simulink model "dvoupatrak_15lan"  (R2019b)
settings: Solver=VariableStepAuto  StartTime=0.0  StopTime=sim_time  RelTol=1e-3  AbsTol=1e-3
InitFcn:
  | parameters_dvoupatrak;
values from neighbouring files (symbols this model uses):
  b_d = b_diameter * ones(6,1)    [parameters_dvoupatrak.m]
  b_l = b_length * ones(6,1)    [parameters_dvoupatrak.m]
  b_rho = b_density * ones(6,1)    [parameters_dvoupatrak.m]
  bp = bpi * ones(15,1)    [parameters_dvoupatrak.m]
  bs = c_specific_damping * ones(15,1)    [parameters_dvoupatrak.m]
  kp = kpi * ones(15,1)    [parameters_dvoupatrak.m]
  ks = c_specific_stiffness * ones(15,1)    [parameters_dvoupatrak.m]
  l0_init = cable_length(node_coords, incidence_table(7:end,:))    [parameters_dvoupatrak.m]
  N = node_coords    [parameters_dvoupatrak.m]
  prestress_cab = 0.95    [simulate.m]
  r_mid = 0.15    [parameters_dvoupatrak.m]
  settling_time = 0.5    [simulate.m]
  sim_time = 5    [simulate.m]
  v1 = sqrt(b_length^2 - (xB-xA)^2 - (yB-yA)^2)    [parameters_dvoupatrak.m]
  v2 = sqrt(b_length^2 - (xC-xB)^2 - (yC-yB)^2)    [parameters_dvoupatrak.m]
undefined symbols (not defined in the file or in its folder): X, Y, Z
libraries: nesl_utility x88, sm_lib x70, cstblocks x15, simulink x8
(part 3 of 4)

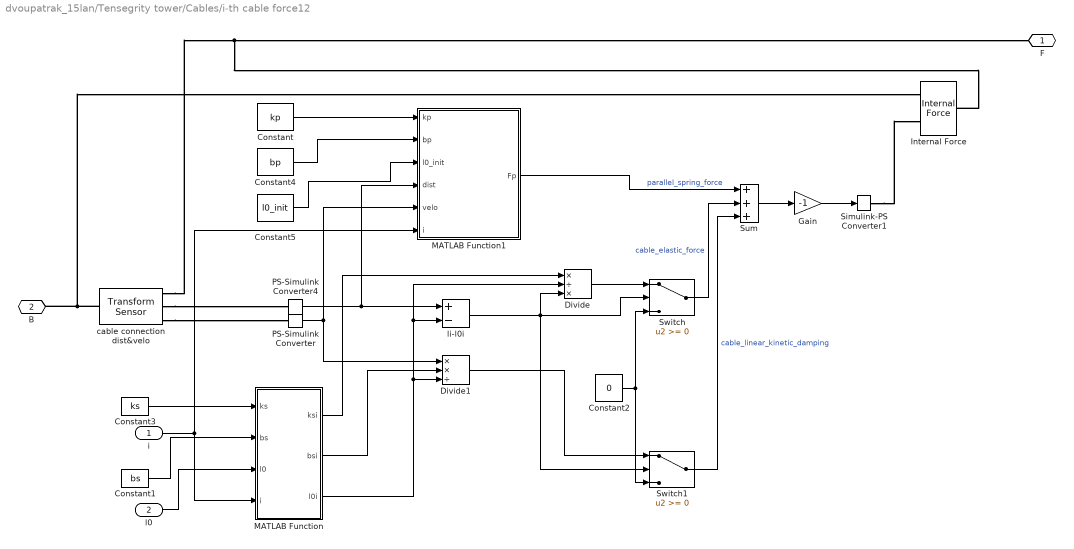
== system dvoupatrak_15lan/Tensegrity tower/Cables/i-th cable force12 ==
  i : Inport
  l0 : Inport  Port=2
  Constant : Constant  Value=kp
  Constant1 : Constant  Value=bs
  Constant2 : Constant  Value=0
  Constant3 : Constant  Value=ks
  Constant4 : Constant  Value=bp
  Constant5 : Constant  Value=l0_init
  Divide : Product  Inputs=*/*
  Divide1 : Product  Inputs=**/
  Gain : Gain  Gain=-1
  Internal Force : sm_lib/Forces and Torques/Internal Force
      settings: SourceProductBaseCode=MS
  MATLAB Function : MATLAB Function  TreatAsAtomicUnit=on
  MATLAB Function1 : MATLAB Function  TreatAsAtomicUnit=on
  PS-Simulink Converter : nesl_utility/PS-Simulink Converter  PhysicalDomain=network_engine_domain  SubClassName=ps_output  LeftPortType=input  RightPortType=output  PseudoPeriodic=off  Frequencies=[]  Unit=inherit  AffineConversion=off
  PS-Simulink Converter4 : nesl_utility/PS-Simulink Converter  PhysicalDomain=network_engine_domain  SubClassName=ps_output  LeftPortType=input  RightPortType=output  PseudoPeriodic=off  Frequencies=[]  Unit=inherit  AffineConversion=off
  Simulink-PS Converter1 : nesl_utility/Simulink-PS Converter  PhysicalDomain=network_engine_domain  SubClassName=ps_input  LeftPortType=input  RightPortType=output  PseudoPeriodic=off  Frequencies=[]  NoiseDistribution=none  NoiseParameters=[]  Unit=1  AffineConversion=off  FilteringAndDerivatives=provide  SimscapeFilterOrder=1  InputFilterTimeConstant=0.001  UdotUserProvided=0
  Sum : Sum  Inputs=+++
  Switch : Switch
  Switch1 : Switch
  cable connection dist&velo : sm_lib/Frames and Transforms/Transform Sensor  MeasurementFrame=World  SenseAngle=off  SenseAxis=off  SenseAngle1=off  SenseAngle2=off  SenseAngle3=off  SenseQ=off  SenseR=off  SenseOmegaX=off  SenseOmegaY=off  SenseOmegaZ=off  SenseOmega1=off  SenseOmega2=off  SenseOmega3=off  SenseQDot=off  SenseRDot=off  SenseAlphaX=off  SenseAlphaY=off  SenseAlphaZ=off  SenseAlpha1=off  SenseAlpha2=off  SenseAlpha3=off  SenseQDDot=off  SenseRDDot=off  SenseX=off  SenseY=off  SenseZ=off  SenseRad=off  SenseAzim=off  SenseDist=on  SenseInc=off  SenseXDot=off  SenseYDot=off  SenseZDot=off  SenseRadDot=off  SenseAzimDot=off  SenseDistDot=on  SenseIncDot=off  SenseXDDot=off  SenseYDDot=off  SenseZDDot=off  SenseRadDDot=off  SenseAzimDDot=off  SenseDistDDot=off  SenseIncDDot=off
  li-l0i : Sum  Inputs=+-
  F : PMIOPort  Side=Right
  B : PMIOPort  Port=2  Side=Left
  wires:
  Constant1/1 -> MATLAB Function/2(bs)
  Switch1/1 -> Sum/3  "cable_linear_kinetic_damping"
  Divide/1 -> Switch/1
  Switch/1 -> Sum/2  "cable_elastic_force"
  MATLAB Function/2(bsi) -> Divide1/2
  Constant3/1 -> MATLAB Function/1(ks)
  Divide1/1 -> Switch1/1
  MATLAB Function/1(ksi) -> Divide/1
  Constant/1 -> MATLAB Function1/1(kp)
  Constant4/1 -> MATLAB Function1/2(bp)
  Constant5/1 -> MATLAB Function1/3(l0_init)
  MATLAB Function1/1(Fp) -> Sum/1  "parallel_spring_force"
  Sum/1 -> Gain/1
  Gain/1 -> Simulink-PS Converter1/1
  li-l0i/1 -> Switch/2, Divide/3, Switch1/2
  l0/1 -> MATLAB Function/3(l0)
  Constant2/1 -> Switch1/3, Switch/3
  MATLAB Function/3(l0i) -> Divide1/3, Divide/2, li-l0i/2
  PS-Simulink Converter4/1 -> li-l0i/1, MATLAB Function1/4(dist)
  PS-Simulink Converter/1 -> Divide1/1, MATLAB Function1/5(velo)
  i/1 -> MATLAB Function/4(i), MATLAB Function1/6(i)
  connections:
  cable connection dist&velo/RConn3 -- PS-Simulink Converter/LConn1
  cable connection dist&velo/RConn1 -- Internal Force/RConn1 -- F/RConn1
  cable connection dist&velo/RConn2 -- PS-Simulink Converter4/LConn1
  Simulink-PS Converter1/RConn1 -- Internal Force/LConn2
  cable connection dist&velo/LConn1 -- B/RConn1 -- Internal Force/LConn1

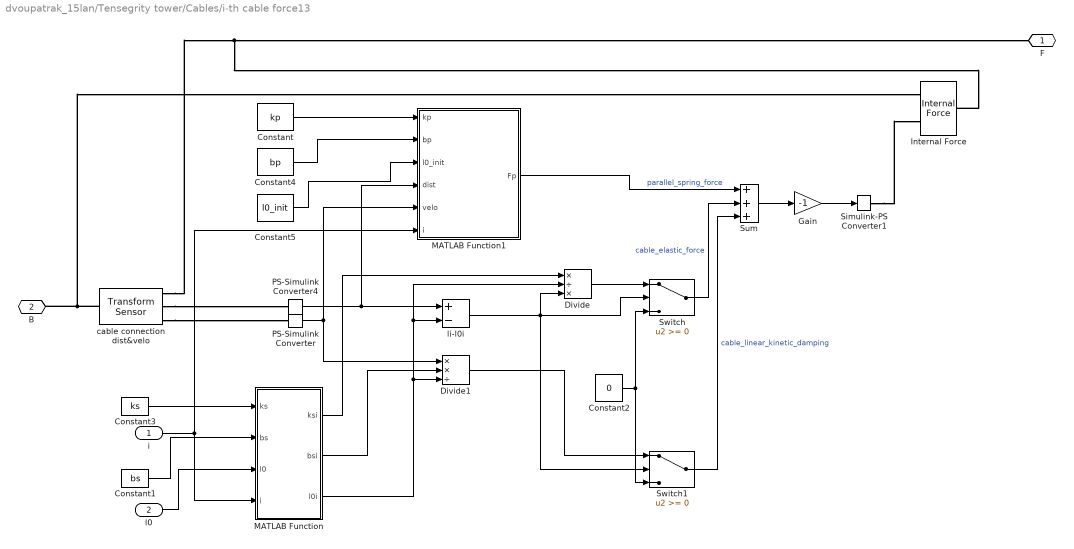
== system dvoupatrak_15lan/Tensegrity tower/Cables/i-th cable force13 ==
  i : Inport
  l0 : Inport  Port=2
  Constant : Constant  Value=kp
  Constant1 : Constant  Value=bs
  Constant2 : Constant  Value=0
  Constant3 : Constant  Value=ks
  Constant4 : Constant  Value=bp
  Constant5 : Constant  Value=l0_init
  Divide : Product  Inputs=*/*
  Divide1 : Product  Inputs=**/
  Gain : Gain  Gain=-1
  Internal Force : sm_lib/Forces and Torques/Internal Force
      settings: SourceProductBaseCode=MS
  MATLAB Function : MATLAB Function  TreatAsAtomicUnit=on
  MATLAB Function1 : MATLAB Function  TreatAsAtomicUnit=on
  PS-Simulink Converter : nesl_utility/PS-Simulink Converter  PhysicalDomain=network_engine_domain  SubClassName=ps_output  LeftPortType=input  RightPortType=output  PseudoPeriodic=off  Frequencies=[]  Unit=inherit  AffineConversion=off
  PS-Simulink Converter4 : nesl_utility/PS-Simulink Converter  PhysicalDomain=network_engine_domain  SubClassName=ps_output  LeftPortType=input  RightPortType=output  PseudoPeriodic=off  Frequencies=[]  Unit=inherit  AffineConversion=off
  Simulink-PS Converter1 : nesl_utility/Simulink-PS Converter  PhysicalDomain=network_engine_domain  SubClassName=ps_input  LeftPortType=input  RightPortType=output  PseudoPeriodic=off  Frequencies=[]  NoiseDistribution=none  NoiseParameters=[]  Unit=1  AffineConversion=off  FilteringAndDerivatives=provide  SimscapeFilterOrder=1  InputFilterTimeConstant=0.001  UdotUserProvided=0
  Sum : Sum  Inputs=+++
  Switch : Switch
  Switch1 : Switch
  cable connection dist&velo : sm_lib/Frames and Transforms/Transform Sensor  MeasurementFrame=World  SenseAngle=off  SenseAxis=off  SenseAngle1=off  SenseAngle2=off  SenseAngle3=off  SenseQ=off  SenseR=off  SenseOmegaX=off  SenseOmegaY=off  SenseOmegaZ=off  SenseOmega1=off  SenseOmega2=off  SenseOmega3=off  SenseQDot=off  SenseRDot=off  SenseAlphaX=off  SenseAlphaY=off  SenseAlphaZ=off  SenseAlpha1=off  SenseAlpha2=off  SenseAlpha3=off  SenseQDDot=off  SenseRDDot=off  SenseX=off  SenseY=off  SenseZ=off  SenseRad=off  SenseAzim=off  SenseDist=on  SenseInc=off  SenseXDot=off  SenseYDot=off  SenseZDot=off  SenseRadDot=off  SenseAzimDot=off  SenseDistDot=on  SenseIncDot=off  SenseXDDot=off  SenseYDDot=off  SenseZDDot=off  SenseRadDDot=off  SenseAzimDDot=off  SenseDistDDot=off  SenseIncDDot=off
  li-l0i : Sum  Inputs=+-
  F : PMIOPort  Side=Right
  B : PMIOPort  Port=2  Side=Left
  wires:
  Constant1/1 -> MATLAB Function/2(bs)
  Switch1/1 -> Sum/3  "cable_linear_kinetic_damping"
  Divide/1 -> Switch/1
  Switch/1 -> Sum/2  "cable_elastic_force"
  MATLAB Function/2(bsi) -> Divide1/2
  Constant3/1 -> MATLAB Function/1(ks)
  Divide1/1 -> Switch1/1
  MATLAB Function/1(ksi) -> Divide/1
  Constant/1 -> MATLAB Function1/1(kp)
  Constant4/1 -> MATLAB Function1/2(bp)
  Constant5/1 -> MATLAB Function1/3(l0_init)
  MATLAB Function1/1(Fp) -> Sum/1  "parallel_spring_force"
  Sum/1 -> Gain/1
  Gain/1 -> Simulink-PS Converter1/1
  li-l0i/1 -> Switch/2, Divide/3, Switch1/2
  l0/1 -> MATLAB Function/3(l0)
  Constant2/1 -> Switch1/3, Switch/3
  MATLAB Function/3(l0i) -> Divide1/3, Divide/2, li-l0i/2
  PS-Simulink Converter4/1 -> li-l0i/1, MATLAB Function1/4(dist)
  PS-Simulink Converter/1 -> Divide1/1, MATLAB Function1/5(velo)
  i/1 -> MATLAB Function/4(i), MATLAB Function1/6(i)
  connections:
  cable connection dist&velo/RConn3 -- PS-Simulink Converter/LConn1
  cable connection dist&velo/RConn1 -- Internal Force/RConn1 -- F/RConn1
  cable connection dist&velo/RConn2 -- PS-Simulink Converter4/LConn1
  Simulink-PS Converter1/RConn1 -- Internal Force/LConn2
  cable connection dist&velo/LConn1 -- B/RConn1 -- Internal Force/LConn1

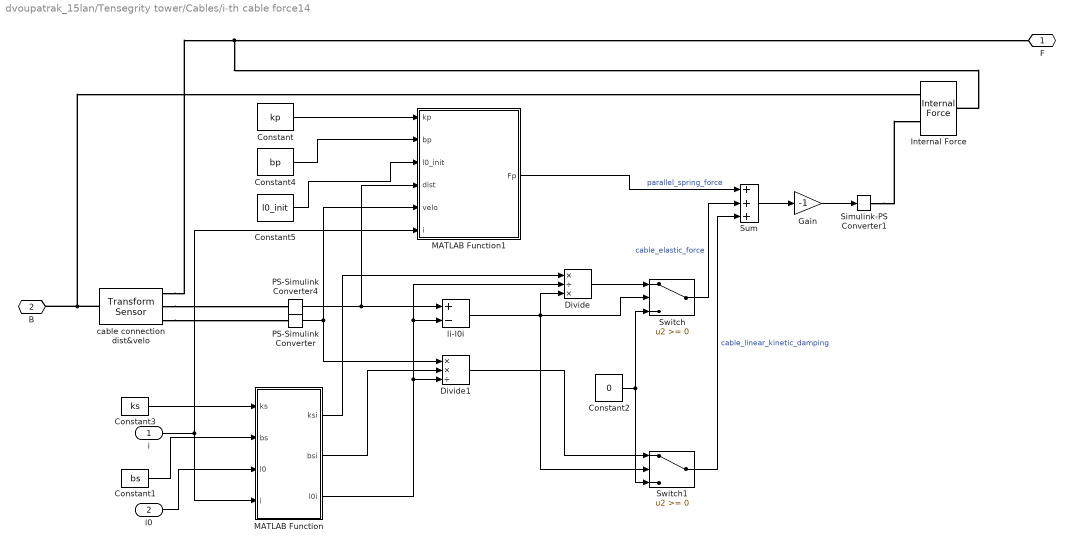
== system dvoupatrak_15lan/Tensegrity tower/Cables/i-th cable force14 ==
  i : Inport
  l0 : Inport  Port=2
  Constant : Constant  Value=kp
  Constant1 : Constant  Value=bs
  Constant2 : Constant  Value=0
  Constant3 : Constant  Value=ks
  Constant4 : Constant  Value=bp
  Constant5 : Constant  Value=l0_init
  Divide : Product  Inputs=*/*
  Divide1 : Product  Inputs=**/
  Gain : Gain  Gain=-1
  Internal Force : sm_lib/Forces and Torques/Internal Force
      settings: SourceProductBaseCode=MS
  MATLAB Function : MATLAB Function  TreatAsAtomicUnit=on
  MATLAB Function1 : MATLAB Function  TreatAsAtomicUnit=on
  PS-Simulink Converter : nesl_utility/PS-Simulink Converter  PhysicalDomain=network_engine_domain  SubClassName=ps_output  LeftPortType=input  RightPortType=output  PseudoPeriodic=off  Frequencies=[]  Unit=inherit  AffineConversion=off
  PS-Simulink Converter4 : nesl_utility/PS-Simulink Converter  PhysicalDomain=network_engine_domain  SubClassName=ps_output  LeftPortType=input  RightPortType=output  PseudoPeriodic=off  Frequencies=[]  Unit=inherit  AffineConversion=off
  Simulink-PS Converter1 : nesl_utility/Simulink-PS Converter  PhysicalDomain=network_engine_domain  SubClassName=ps_input  LeftPortType=input  RightPortType=output  PseudoPeriodic=off  Frequencies=[]  NoiseDistribution=none  NoiseParameters=[]  Unit=1  AffineConversion=off  FilteringAndDerivatives=provide  SimscapeFilterOrder=1  InputFilterTimeConstant=0.001  UdotUserProvided=0
  Sum : Sum  Inputs=+++
  Switch : Switch
  Switch1 : Switch
  cable connection dist&velo : sm_lib/Frames and Transforms/Transform Sensor  MeasurementFrame=World  SenseAngle=off  SenseAxis=off  SenseAngle1=off  SenseAngle2=off  SenseAngle3=off  SenseQ=off  SenseR=off  SenseOmegaX=off  SenseOmegaY=off  SenseOmegaZ=off  SenseOmega1=off  SenseOmega2=off  SenseOmega3=off  SenseQDot=off  SenseRDot=off  SenseAlphaX=off  SenseAlphaY=off  SenseAlphaZ=off  SenseAlpha1=off  SenseAlpha2=off  SenseAlpha3=off  SenseQDDot=off  SenseRDDot=off  SenseX=off  SenseY=off  SenseZ=off  SenseRad=off  SenseAzim=off  SenseDist=on  SenseInc=off  SenseXDot=off  SenseYDot=off  SenseZDot=off  SenseRadDot=off  SenseAzimDot=off  SenseDistDot=on  SenseIncDot=off  SenseXDDot=off  SenseYDDot=off  SenseZDDot=off  SenseRadDDot=off  SenseAzimDDot=off  SenseDistDDot=off  SenseIncDDot=off
  li-l0i : Sum  Inputs=+-
  F : PMIOPort  Side=Right
  B : PMIOPort  Port=2  Side=Left
  wires:
  Constant1/1 -> MATLAB Function/2(bs)
  Switch1/1 -> Sum/3  "cable_linear_kinetic_damping"
  Divide/1 -> Switch/1
  Switch/1 -> Sum/2  "cable_elastic_force"
  MATLAB Function/2(bsi) -> Divide1/2
  Constant3/1 -> MATLAB Function/1(ks)
  Divide1/1 -> Switch1/1
  MATLAB Function/1(ksi) -> Divide/1
  Constant/1 -> MATLAB Function1/1(kp)
  Constant4/1 -> MATLAB Function1/2(bp)
  Constant5/1 -> MATLAB Function1/3(l0_init)
  MATLAB Function1/1(Fp) -> Sum/1  "parallel_spring_force"
  Sum/1 -> Gain/1
  Gain/1 -> Simulink-PS Converter1/1
  li-l0i/1 -> Switch/2, Divide/3, Switch1/2
  l0/1 -> MATLAB Function/3(l0)
  Constant2/1 -> Switch1/3, Switch/3
  MATLAB Function/3(l0i) -> Divide1/3, Divide/2, li-l0i/2
  PS-Simulink Converter4/1 -> li-l0i/1, MATLAB Function1/4(dist)
  PS-Simulink Converter/1 -> Divide1/1, MATLAB Function1/5(velo)
  i/1 -> MATLAB Function/4(i), MATLAB Function1/6(i)
  connections:
  cable connection dist&velo/RConn3 -- PS-Simulink Converter/LConn1
  cable connection dist&velo/RConn1 -- Internal Force/RConn1 -- F/RConn1
  cable connection dist&velo/RConn2 -- PS-Simulink Converter4/LConn1
  Simulink-PS Converter1/RConn1 -- Internal Force/LConn2
  cable connection dist&velo/LConn1 -- B/RConn1 -- Internal Force/LConn1

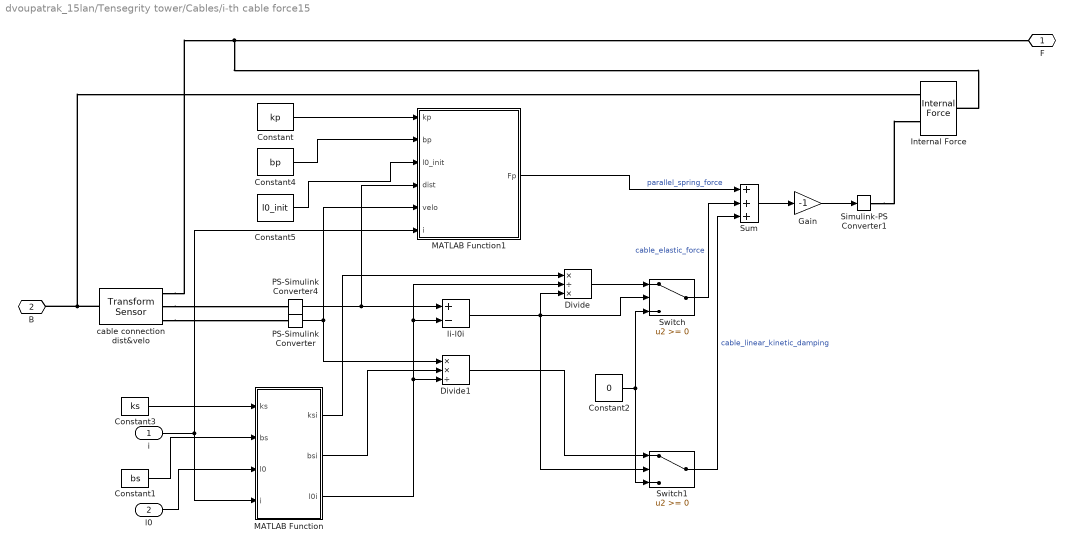
== system dvoupatrak_15lan/Tensegrity tower/Cables/i-th cable force15 ==
  i : Inport
  l0 : Inport  Port=2
  Constant : Constant  Value=kp
  Constant1 : Constant  Value=bs
  Constant2 : Constant  Value=0
  Constant3 : Constant  Value=ks
  Constant4 : Constant  Value=bp
  Constant5 : Constant  Value=l0_init
  Divide : Product  Inputs=*/*
  Divide1 : Product  Inputs=**/
  Gain : Gain  Gain=-1
  Internal Force : sm_lib/Forces and Torques/Internal Force
      settings: SourceProductBaseCode=MS
  MATLAB Function : MATLAB Function  TreatAsAtomicUnit=on
  MATLAB Function1 : MATLAB Function  TreatAsAtomicUnit=on
  PS-Simulink Converter : nesl_utility/PS-Simulink Converter  PhysicalDomain=network_engine_domain  SubClassName=ps_output  LeftPortType=input  RightPortType=output  PseudoPeriodic=off  Frequencies=[]  Unit=inherit  AffineConversion=off
  PS-Simulink Converter4 : nesl_utility/PS-Simulink Converter  PhysicalDomain=network_engine_domain  SubClassName=ps_output  LeftPortType=input  RightPortType=output  PseudoPeriodic=off  Frequencies=[]  Unit=inherit  AffineConversion=off
  Simulink-PS Converter1 : nesl_utility/Simulink-PS Converter  PhysicalDomain=network_engine_domain  SubClassName=ps_input  LeftPortType=input  RightPortType=output  PseudoPeriodic=off  Frequencies=[]  NoiseDistribution=none  NoiseParameters=[]  Unit=1  AffineConversion=off  FilteringAndDerivatives=provide  SimscapeFilterOrder=1  InputFilterTimeConstant=0.001  UdotUserProvided=0
  Sum : Sum  Inputs=+++
  Switch : Switch
  Switch1 : Switch
  cable connection dist&velo : sm_lib/Frames and Transforms/Transform Sensor  MeasurementFrame=World  SenseAngle=off  SenseAxis=off  SenseAngle1=off  SenseAngle2=off  SenseAngle3=off  SenseQ=off  SenseR=off  SenseOmegaX=off  SenseOmegaY=off  SenseOmegaZ=off  SenseOmega1=off  SenseOmega2=off  SenseOmega3=off  SenseQDot=off  SenseRDot=off  SenseAlphaX=off  SenseAlphaY=off  SenseAlphaZ=off  SenseAlpha1=off  SenseAlpha2=off  SenseAlpha3=off  SenseQDDot=off  SenseRDDot=off  SenseX=off  SenseY=off  SenseZ=off  SenseRad=off  SenseAzim=off  SenseDist=on  SenseInc=off  SenseXDot=off  SenseYDot=off  SenseZDot=off  SenseRadDot=off  SenseAzimDot=off  SenseDistDot=on  SenseIncDot=off  SenseXDDot=off  SenseYDDot=off  SenseZDDot=off  SenseRadDDot=off  SenseAzimDDot=off  SenseDistDDot=off  SenseIncDDot=off
  li-l0i : Sum  Inputs=+-
  F : PMIOPort  Side=Right
  B : PMIOPort  Port=2  Side=Left
  wires:
  Constant1/1 -> MATLAB Function/2(bs)
  Switch1/1 -> Sum/3  "cable_linear_kinetic_damping"
  Divide/1 -> Switch/1
  Switch/1 -> Sum/2  "cable_elastic_force"
  MATLAB Function/2(bsi) -> Divide1/2
  Constant3/1 -> MATLAB Function/1(ks)
  Divide1/1 -> Switch1/1
  MATLAB Function/1(ksi) -> Divide/1
  Constant/1 -> MATLAB Function1/1(kp)
  Constant4/1 -> MATLAB Function1/2(bp)
  Constant5/1 -> MATLAB Function1/3(l0_init)
  MATLAB Function1/1(Fp) -> Sum/1  "parallel_spring_force"
  Sum/1 -> Gain/1
  Gain/1 -> Simulink-PS Converter1/1
  li-l0i/1 -> Switch/2, Divide/3, Switch1/2
  l0/1 -> MATLAB Function/3(l0)
  Constant2/1 -> Switch1/3, Switch/3
  MATLAB Function/3(l0i) -> Divide1/3, Divide/2, li-l0i/2
  PS-Simulink Converter4/1 -> li-l0i/1, MATLAB Function1/4(dist)
  PS-Simulink Converter/1 -> Divide1/1, MATLAB Function1/5(velo)
  i/1 -> MATLAB Function/4(i), MATLAB Function1/6(i)
  connections:
  cable connection dist&velo/RConn3 -- PS-Simulink Converter/LConn1
  cable connection dist&velo/RConn1 -- Internal Force/RConn1 -- F/RConn1
  cable connection dist&velo/RConn2 -- PS-Simulink Converter4/LConn1
  Simulink-PS Converter1/RConn1 -- Internal Force/LConn2
  cable connection dist&velo/LConn1 -- B/RConn1 -- Internal Force/LConn1

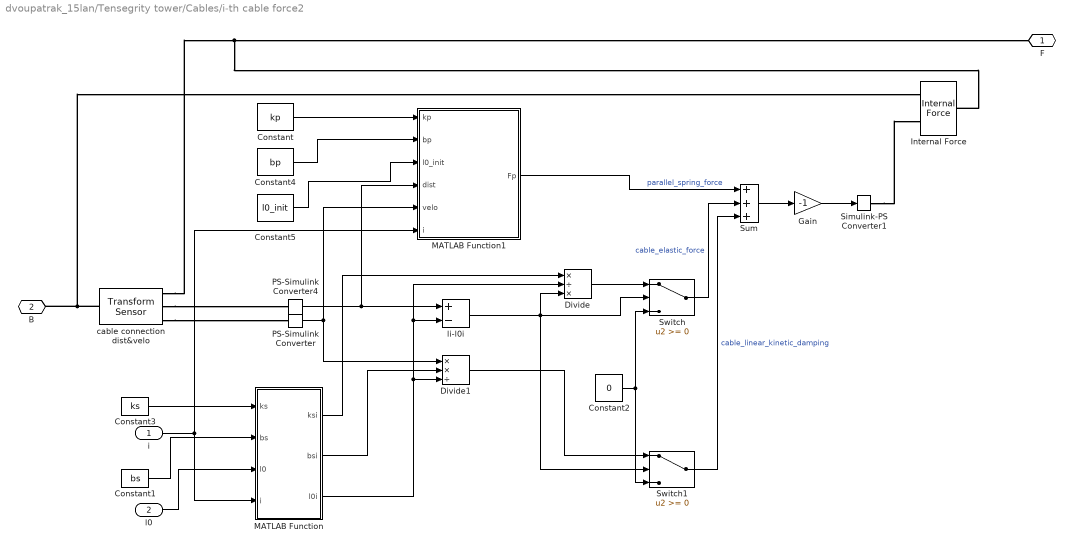
== system dvoupatrak_15lan/Tensegrity tower/Cables/i-th cable force2 ==
  i : Inport
  l0 : Inport  Port=2
  Constant : Constant  Value=kp
  Constant1 : Constant  Value=bs
  Constant2 : Constant  Value=0
  Constant3 : Constant  Value=ks
  Constant4 : Constant  Value=bp
  Constant5 : Constant  Value=l0_init
  Divide : Product  Inputs=*/*
  Divide1 : Product  Inputs=**/
  Gain : Gain  Gain=-1
  Internal Force : sm_lib/Forces and Torques/Internal Force
      settings: SourceProductBaseCode=MS
  MATLAB Function : MATLAB Function  TreatAsAtomicUnit=on
  MATLAB Function1 : MATLAB Function  TreatAsAtomicUnit=on
  PS-Simulink Converter : nesl_utility/PS-Simulink Converter  PhysicalDomain=network_engine_domain  SubClassName=ps_output  LeftPortType=input  RightPortType=output  PseudoPeriodic=off  Frequencies=[]  Unit=inherit  AffineConversion=off
  PS-Simulink Converter4 : nesl_utility/PS-Simulink Converter  PhysicalDomain=network_engine_domain  SubClassName=ps_output  LeftPortType=input  RightPortType=output  PseudoPeriodic=off  Frequencies=[]  Unit=inherit  AffineConversion=off
  Simulink-PS Converter1 : nesl_utility/Simulink-PS Converter  PhysicalDomain=network_engine_domain  SubClassName=ps_input  LeftPortType=input  RightPortType=output  PseudoPeriodic=off  Frequencies=[]  NoiseDistribution=none  NoiseParameters=[]  Unit=1  AffineConversion=off  FilteringAndDerivatives=provide  SimscapeFilterOrder=1  InputFilterTimeConstant=0.001  UdotUserProvided=0
  Sum : Sum  Inputs=+++
  Switch : Switch
  Switch1 : Switch
  cable connection dist&velo : sm_lib/Frames and Transforms/Transform Sensor  MeasurementFrame=World  SenseAngle=off  SenseAxis=off  SenseAngle1=off  SenseAngle2=off  SenseAngle3=off  SenseQ=off  SenseR=off  SenseOmegaX=off  SenseOmegaY=off  SenseOmegaZ=off  SenseOmega1=off  SenseOmega2=off  SenseOmega3=off  SenseQDot=off  SenseRDot=off  SenseAlphaX=off  SenseAlphaY=off  SenseAlphaZ=off  SenseAlpha1=off  SenseAlpha2=off  SenseAlpha3=off  SenseQDDot=off  SenseRDDot=off  SenseX=off  SenseY=off  SenseZ=off  SenseRad=off  SenseAzim=off  SenseDist=on  SenseInc=off  SenseXDot=off  SenseYDot=off  SenseZDot=off  SenseRadDot=off  SenseAzimDot=off  SenseDistDot=on  SenseIncDot=off  SenseXDDot=off  SenseYDDot=off  SenseZDDot=off  SenseRadDDot=off  SenseAzimDDot=off  SenseDistDDot=off  SenseIncDDot=off
  li-l0i : Sum  Inputs=+-
  F : PMIOPort  Side=Right
  B : PMIOPort  Port=2  Side=Left
  wires:
  Constant1/1 -> MATLAB Function/2(bs)
  Switch1/1 -> Sum/3  "cable_linear_kinetic_damping"
  Divide/1 -> Switch/1
  Switch/1 -> Sum/2  "cable_elastic_force"
  MATLAB Function/2(bsi) -> Divide1/2
  Constant3/1 -> MATLAB Function/1(ks)
  Divide1/1 -> Switch1/1
  MATLAB Function/1(ksi) -> Divide/1
  Constant/1 -> MATLAB Function1/1(kp)
  Constant4/1 -> MATLAB Function1/2(bp)
  Constant5/1 -> MATLAB Function1/3(l0_init)
  MATLAB Function1/1(Fp) -> Sum/1  "parallel_spring_force"
  Sum/1 -> Gain/1
  Gain/1 -> Simulink-PS Converter1/1
  li-l0i/1 -> Switch/2, Divide/3, Switch1/2
  l0/1 -> MATLAB Function/3(l0)
  Constant2/1 -> Switch1/3, Switch/3
  MATLAB Function/3(l0i) -> Divide1/3, Divide/2, li-l0i/2
  PS-Simulink Converter4/1 -> li-l0i/1, MATLAB Function1/4(dist)
  PS-Simulink Converter/1 -> Divide1/1, MATLAB Function1/5(velo)
  i/1 -> MATLAB Function/4(i), MATLAB Function1/6(i)
  connections:
  cable connection dist&velo/RConn3 -- PS-Simulink Converter/LConn1
  cable connection dist&velo/RConn1 -- Internal Force/RConn1 -- F/RConn1
  cable connection dist&velo/RConn2 -- PS-Simulink Converter4/LConn1
  Simulink-PS Converter1/RConn1 -- Internal Force/LConn2
  cable connection dist&velo/LConn1 -- B/RConn1 -- Internal Force/LConn1

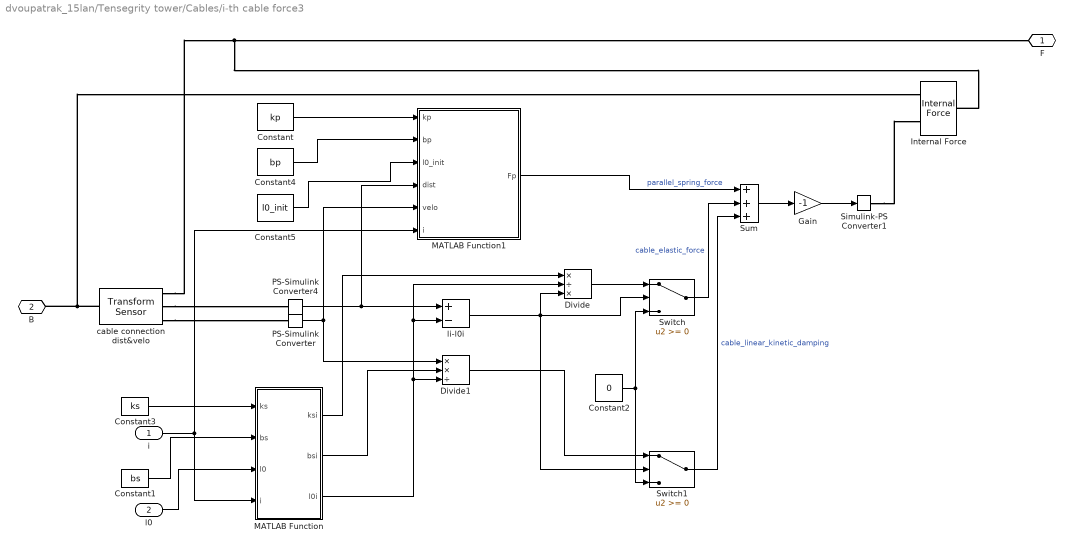
== system dvoupatrak_15lan/Tensegrity tower/Cables/i-th cable force3 ==
  i : Inport
  l0 : Inport  Port=2
  Constant : Constant  Value=kp
  Constant1 : Constant  Value=bs
  Constant2 : Constant  Value=0
  Constant3 : Constant  Value=ks
  Constant4 : Constant  Value=bp
  Constant5 : Constant  Value=l0_init
  Divide : Product  Inputs=*/*
  Divide1 : Product  Inputs=**/
  Gain : Gain  Gain=-1
  Internal Force : sm_lib/Forces and Torques/Internal Force
      settings: SourceProductBaseCode=MS
  MATLAB Function : MATLAB Function  TreatAsAtomicUnit=on
  MATLAB Function1 : MATLAB Function  TreatAsAtomicUnit=on
  PS-Simulink Converter : nesl_utility/PS-Simulink Converter  PhysicalDomain=network_engine_domain  SubClassName=ps_output  LeftPortType=input  RightPortType=output  PseudoPeriodic=off  Frequencies=[]  Unit=inherit  AffineConversion=off
  PS-Simulink Converter4 : nesl_utility/PS-Simulink Converter  PhysicalDomain=network_engine_domain  SubClassName=ps_output  LeftPortType=input  RightPortType=output  PseudoPeriodic=off  Frequencies=[]  Unit=inherit  AffineConversion=off
  Simulink-PS Converter1 : nesl_utility/Simulink-PS Converter  PhysicalDomain=network_engine_domain  SubClassName=ps_input  LeftPortType=input  RightPortType=output  PseudoPeriodic=off  Frequencies=[]  NoiseDistribution=none  NoiseParameters=[]  Unit=1  AffineConversion=off  FilteringAndDerivatives=provide  SimscapeFilterOrder=1  InputFilterTimeConstant=0.001  UdotUserProvided=0
  Sum : Sum  Inputs=+++
  Switch : Switch
  Switch1 : Switch
  cable connection dist&velo : sm_lib/Frames and Transforms/Transform Sensor  MeasurementFrame=World  SenseAngle=off  SenseAxis=off  SenseAngle1=off  SenseAngle2=off  SenseAngle3=off  SenseQ=off  SenseR=off  SenseOmegaX=off  SenseOmegaY=off  SenseOmegaZ=off  SenseOmega1=off  SenseOmega2=off  SenseOmega3=off  SenseQDot=off  SenseRDot=off  SenseAlphaX=off  SenseAlphaY=off  SenseAlphaZ=off  SenseAlpha1=off  SenseAlpha2=off  SenseAlpha3=off  SenseQDDot=off  SenseRDDot=off  SenseX=off  SenseY=off  SenseZ=off  SenseRad=off  SenseAzim=off  SenseDist=on  SenseInc=off  SenseXDot=off  SenseYDot=off  SenseZDot=off  SenseRadDot=off  SenseAzimDot=off  SenseDistDot=on  SenseIncDot=off  SenseXDDot=off  SenseYDDot=off  SenseZDDot=off  SenseRadDDot=off  SenseAzimDDot=off  SenseDistDDot=off  SenseIncDDot=off
  li-l0i : Sum  Inputs=+-
  F : PMIOPort  Side=Right
  B : PMIOPort  Port=2  Side=Left
  wires:
  Constant1/1 -> MATLAB Function/2(bs)
  Switch1/1 -> Sum/3  "cable_linear_kinetic_damping"
  Divide/1 -> Switch/1
  Switch/1 -> Sum/2  "cable_elastic_force"
  MATLAB Function/2(bsi) -> Divide1/2
  Constant3/1 -> MATLAB Function/1(ks)
  Divide1/1 -> Switch1/1
  MATLAB Function/1(ksi) -> Divide/1
  Constant/1 -> MATLAB Function1/1(kp)
  Constant4/1 -> MATLAB Function1/2(bp)
  Constant5/1 -> MATLAB Function1/3(l0_init)
  MATLAB Function1/1(Fp) -> Sum/1  "parallel_spring_force"
  Sum/1 -> Gain/1
  Gain/1 -> Simulink-PS Converter1/1
  li-l0i/1 -> Switch/2, Divide/3, Switch1/2
  l0/1 -> MATLAB Function/3(l0)
  Constant2/1 -> Switch1/3, Switch/3
  MATLAB Function/3(l0i) -> Divide1/3, Divide/2, li-l0i/2
  PS-Simulink Converter4/1 -> li-l0i/1, MATLAB Function1/4(dist)
  PS-Simulink Converter/1 -> Divide1/1, MATLAB Function1/5(velo)
  i/1 -> MATLAB Function/4(i), MATLAB Function1/6(i)
  connections:
  cable connection dist&velo/RConn3 -- PS-Simulink Converter/LConn1
  cable connection dist&velo/RConn1 -- Internal Force/RConn1 -- F/RConn1
  cable connection dist&velo/RConn2 -- PS-Simulink Converter4/LConn1
  Simulink-PS Converter1/RConn1 -- Internal Force/LConn2
  cable connection dist&velo/LConn1 -- B/RConn1 -- Internal Force/LConn1

== system dvoupatrak_15lan/Tensegrity tower/Cables/i-th cable force4 ==
  i : Inport
  l0 : Inport  Port=2
  Constant : Constant  Value=kp
  Constant1 : Constant  Value=bs
  Constant2 : Constant  Value=0
  Constant3 : Constant  Value=ks
  Constant4 : Constant  Value=bp
  Constant5 : Constant  Value=l0_init
  Divide : Product  Inputs=*/*
  Divide1 : Product  Inputs=**/
  Gain : Gain  Gain=-1
  Internal Force : sm_lib/Forces and Torques/Internal Force
      settings: SourceProductBaseCode=MS
  MATLAB Function : MATLAB Function  TreatAsAtomicUnit=on
  MATLAB Function1 : MATLAB Function  TreatAsAtomicUnit=on
  PS-Simulink Converter : nesl_utility/PS-Simulink Converter  PhysicalDomain=network_engine_domain  SubClassName=ps_output  LeftPortType=input  RightPortType=output  PseudoPeriodic=off  Frequencies=[]  Unit=inherit  AffineConversion=off
  PS-Simulink Converter4 : nesl_utility/PS-Simulink Converter  PhysicalDomain=network_engine_domain  SubClassName=ps_output  LeftPortType=input  RightPortType=output  PseudoPeriodic=off  Frequencies=[]  Unit=inherit  AffineConversion=off
  Simulink-PS Converter1 : nesl_utility/Simulink-PS Converter  PhysicalDomain=network_engine_domain  SubClassName=ps_input  LeftPortType=input  RightPortType=output  PseudoPeriodic=off  Frequencies=[]  NoiseDistribution=none  NoiseParameters=[]  Unit=1  AffineConversion=off  FilteringAndDerivatives=provide  SimscapeFilterOrder=1  InputFilterTimeConstant=0.001  UdotUserProvided=0
  Sum : Sum  Inputs=+++
  Switch : Switch
  Switch1 : Switch
  cable connection dist&velo : sm_lib/Frames and Transforms/Transform Sensor  MeasurementFrame=World  SenseAngle=off  SenseAxis=off  SenseAngle1=off  SenseAngle2=off  SenseAngle3=off  SenseQ=off  SenseR=off  SenseOmegaX=off  SenseOmegaY=off  SenseOmegaZ=off  SenseOmega1=off  SenseOmega2=off  SenseOmega3=off  SenseQDot=off  SenseRDot=off  SenseAlphaX=off  SenseAlphaY=off  SenseAlphaZ=off  SenseAlpha1=off  SenseAlpha2=off  SenseAlpha3=off  SenseQDDot=off  SenseRDDot=off  SenseX=off  SenseY=off  SenseZ=off  SenseRad=off  SenseAzim=off  SenseDist=on  SenseInc=off  SenseXDot=off  SenseYDot=off  SenseZDot=off  SenseRadDot=off  SenseAzimDot=off  SenseDistDot=on  SenseIncDot=off  SenseXDDot=off  SenseYDDot=off  SenseZDDot=off  SenseRadDDot=off  SenseAzimDDot=off  SenseDistDDot=off  SenseIncDDot=off
  li-l0i : Sum  Inputs=+-
  F : PMIOPort  Side=Right
  B : PMIOPort  Port=2  Side=Left
  wires:
  Constant1/1 -> MATLAB Function/2(bs)
  Switch1/1 -> Sum/3  "cable_linear_kinetic_damping"
  Divide/1 -> Switch/1
  Switch/1 -> Sum/2  "cable_elastic_force"
  MATLAB Function/2(bsi) -> Divide1/2
  Constant3/1 -> MATLAB Function/1(ks)
  Divide1/1 -> Switch1/1
  MATLAB Function/1(ksi) -> Divide/1
  Constant/1 -> MATLAB Function1/1(kp)
  Constant4/1 -> MATLAB Function1/2(bp)
  Constant5/1 -> MATLAB Function1/3(l0_init)
  MATLAB Function1/1(Fp) -> Sum/1  "parallel_spring_force"
  Sum/1 -> Gain/1
  Gain/1 -> Simulink-PS Converter1/1
  li-l0i/1 -> Switch/2, Divide/3, Switch1/2
  l0/1 -> MATLAB Function/3(l0)
  Constant2/1 -> Switch1/3, Switch/3
  MATLAB Function/3(l0i) -> Divide1/3, Divide/2, li-l0i/2
  PS-Simulink Converter4/1 -> li-l0i/1, MATLAB Function1/4(dist)
  PS-Simulink Converter/1 -> Divide1/1, MATLAB Function1/5(velo)
  i/1 -> MATLAB Function/4(i), MATLAB Function1/6(i)
  connections:
  cable connection dist&velo/RConn3 -- PS-Simulink Converter/LConn1
  cable connection dist&velo/RConn1 -- Internal Force/RConn1 -- F/RConn1
  cable connection dist&velo/RConn2 -- PS-Simulink Converter4/LConn1
  Simulink-PS Converter1/RConn1 -- Internal Force/LConn2
  cable connection dist&velo/LConn1 -- B/RConn1 -- Internal Force/LConn1

== system dvoupatrak_15lan/Tensegrity tower/Cables/i-th cable force5 ==
  i : Inport
  l0 : Inport  Port=2
  Constant : Constant  Value=kp
  Constant1 : Constant  Value=bs
  Constant2 : Constant  Value=0
  Constant3 : Constant  Value=ks
  Constant4 : Constant  Value=bp
  Constant5 : Constant  Value=l0_init
  Divide : Product  Inputs=*/*
  Divide1 : Product  Inputs=**/
  Gain : Gain  Gain=-1
  Internal Force : sm_lib/Forces and Torques/Internal Force
      settings: SourceProductBaseCode=MS
  MATLAB Function : MATLAB Function  TreatAsAtomicUnit=on
  MATLAB Function1 : MATLAB Function  TreatAsAtomicUnit=on
  PS-Simulink Converter : nesl_utility/PS-Simulink Converter  PhysicalDomain=network_engine_domain  SubClassName=ps_output  LeftPortType=input  RightPortType=output  PseudoPeriodic=off  Frequencies=[]  Unit=inherit  AffineConversion=off
  PS-Simulink Converter4 : nesl_utility/PS-Simulink Converter  PhysicalDomain=network_engine_domain  SubClassName=ps_output  LeftPortType=input  RightPortType=output  PseudoPeriodic=off  Frequencies=[]  Unit=inherit  AffineConversion=off
  Simulink-PS Converter1 : nesl_utility/Simulink-PS Converter  PhysicalDomain=network_engine_domain  SubClassName=ps_input  LeftPortType=input  RightPortType=output  PseudoPeriodic=off  Frequencies=[]  NoiseDistribution=none  NoiseParameters=[]  Unit=1  AffineConversion=off  FilteringAndDerivatives=provide  SimscapeFilterOrder=1  InputFilterTimeConstant=0.001  UdotUserProvided=0
  Sum : Sum  Inputs=+++
  Switch : Switch
  Switch1 : Switch
  cable connection dist&velo : sm_lib/Frames and Transforms/Transform Sensor  MeasurementFrame=World  SenseAngle=off  SenseAxis=off  SenseAngle1=off  SenseAngle2=off  SenseAngle3=off  SenseQ=off  SenseR=off  SenseOmegaX=off  SenseOmegaY=off  SenseOmegaZ=off  SenseOmega1=off  SenseOmega2=off  SenseOmega3=off  SenseQDot=off  SenseRDot=off  SenseAlphaX=off  SenseAlphaY=off  SenseAlphaZ=off  SenseAlpha1=off  SenseAlpha2=off  SenseAlpha3=off  SenseQDDot=off  SenseRDDot=off  SenseX=off  SenseY=off  SenseZ=off  SenseRad=off  SenseAzim=off  SenseDist=on  SenseInc=off  SenseXDot=off  SenseYDot=off  SenseZDot=off  SenseRadDot=off  SenseAzimDot=off  SenseDistDot=on  SenseIncDot=off  SenseXDDot=off  SenseYDDot=off  SenseZDDot=off  SenseRadDDot=off  SenseAzimDDot=off  SenseDistDDot=off  SenseIncDDot=off
  li-l0i : Sum  Inputs=+-
  F : PMIOPort  Side=Right
  B : PMIOPort  Port=2  Side=Left
  wires:
  Constant1/1 -> MATLAB Function/2(bs)
  Switch1/1 -> Sum/3  "cable_linear_kinetic_damping"
  Divide/1 -> Switch/1
  Switch/1 -> Sum/2  "cable_elastic_force"
  MATLAB Function/2(bsi) -> Divide1/2
  Constant3/1 -> MATLAB Function/1(ks)
  Divide1/1 -> Switch1/1
  MATLAB Function/1(ksi) -> Divide/1
  Constant/1 -> MATLAB Function1/1(kp)
  Constant4/1 -> MATLAB Function1/2(bp)
  Constant5/1 -> MATLAB Function1/3(l0_init)
  MATLAB Function1/1(Fp) -> Sum/1  "parallel_spring_force"
  Sum/1 -> Gain/1
  Gain/1 -> Simulink-PS Converter1/1
  li-l0i/1 -> Switch/2, Divide/3, Switch1/2
  l0/1 -> MATLAB Function/3(l0)
  Constant2/1 -> Switch1/3, Switch/3
  MATLAB Function/3(l0i) -> Divide1/3, Divide/2, li-l0i/2
  PS-Simulink Converter4/1 -> li-l0i/1, MATLAB Function1/4(dist)
  PS-Simulink Converter/1 -> Divide1/1, MATLAB Function1/5(velo)
  i/1 -> MATLAB Function/4(i), MATLAB Function1/6(i)
  connections:
  cable connection dist&velo/RConn3 -- PS-Simulink Converter/LConn1
  cable connection dist&velo/RConn1 -- Internal Force/RConn1 -- F/RConn1
  cable connection dist&velo/RConn2 -- PS-Simulink Converter4/LConn1
  Simulink-PS Converter1/RConn1 -- Internal Force/LConn2
  cable connection dist&velo/LConn1 -- B/RConn1 -- Internal Force/LConn1

== system dvoupatrak_15lan/Tensegrity tower/Cables/i-th cable force6 ==
  i : Inport
  l0 : Inport  Port=2
  Constant : Constant  Value=kp
  Constant1 : Constant  Value=bs
  Constant2 : Constant  Value=0
  Constant3 : Constant  Value=ks
  Constant4 : Constant  Value=bp
  Constant5 : Constant  Value=l0_init
  Divide : Product  Inputs=*/*
  Divide1 : Product  Inputs=**/
  Gain : Gain  Gain=-1
  Internal Force : sm_lib/Forces and Torques/Internal Force
      settings: SourceProductBaseCode=MS
  MATLAB Function : MATLAB Function  TreatAsAtomicUnit=on
  MATLAB Function1 : MATLAB Function  TreatAsAtomicUnit=on
  PS-Simulink Converter : nesl_utility/PS-Simulink Converter  PhysicalDomain=network_engine_domain  SubClassName=ps_output  LeftPortType=input  RightPortType=output  PseudoPeriodic=off  Frequencies=[]  Unit=inherit  AffineConversion=off
  PS-Simulink Converter4 : nesl_utility/PS-Simulink Converter  PhysicalDomain=network_engine_domain  SubClassName=ps_output  LeftPortType=input  RightPortType=output  PseudoPeriodic=off  Frequencies=[]  Unit=inherit  AffineConversion=off
  Simulink-PS Converter1 : nesl_utility/Simulink-PS Converter  PhysicalDomain=network_engine_domain  SubClassName=ps_input  LeftPortType=input  RightPortType=output  PseudoPeriodic=off  Frequencies=[]  NoiseDistribution=none  NoiseParameters=[]  Unit=1  AffineConversion=off  FilteringAndDerivatives=provide  SimscapeFilterOrder=1  InputFilterTimeConstant=0.001  UdotUserProvided=0
  Sum : Sum  Inputs=+++
  Switch : Switch
  Switch1 : Switch
  cable connection dist&velo : sm_lib/Frames and Transforms/Transform Sensor  MeasurementFrame=World  SenseAngle=off  SenseAxis=off  SenseAngle1=off  SenseAngle2=off  SenseAngle3=off  SenseQ=off  SenseR=off  SenseOmegaX=off  SenseOmegaY=off  SenseOmegaZ=off  SenseOmega1=off  SenseOmega2=off  SenseOmega3=off  SenseQDot=off  SenseRDot=off  SenseAlphaX=off  SenseAlphaY=off  SenseAlphaZ=off  SenseAlpha1=off  SenseAlpha2=off  SenseAlpha3=off  SenseQDDot=off  SenseRDDot=off  SenseX=off  SenseY=off  SenseZ=off  SenseRad=off  SenseAzim=off  SenseDist=on  SenseInc=off  SenseXDot=off  SenseYDot=off  SenseZDot=off  SenseRadDot=off  SenseAzimDot=off  SenseDistDot=on  SenseIncDot=off  SenseXDDot=off  SenseYDDot=off  SenseZDDot=off  SenseRadDDot=off  SenseAzimDDot=off  SenseDistDDot=off  SenseIncDDot=off
  li-l0i : Sum  Inputs=+-
  F : PMIOPort  Side=Right
  B : PMIOPort  Port=2  Side=Left
  wires:
  Constant1/1 -> MATLAB Function/2(bs)
  Switch1/1 -> Sum/3  "cable_linear_kinetic_damping"
  Divide/1 -> Switch/1
  Switch/1 -> Sum/2  "cable_elastic_force"
  MATLAB Function/2(bsi) -> Divide1/2
  Constant3/1 -> MATLAB Function/1(ks)
  Divide1/1 -> Switch1/1
  MATLAB Function/1(ksi) -> Divide/1
  Constant/1 -> MATLAB Function1/1(kp)
  Constant4/1 -> MATLAB Function1/2(bp)
  Constant5/1 -> MATLAB Function1/3(l0_init)
  MATLAB Function1/1(Fp) -> Sum/1  "parallel_spring_force"
  Sum/1 -> Gain/1
  Gain/1 -> Simulink-PS Converter1/1
  li-l0i/1 -> Switch/2, Divide/3, Switch1/2
  l0/1 -> MATLAB Function/3(l0)
  Constant2/1 -> Switch1/3, Switch/3
  MATLAB Function/3(l0i) -> Divide1/3, Divide/2, li-l0i/2
  PS-Simulink Converter4/1 -> li-l0i/1, MATLAB Function1/4(dist)
  PS-Simulink Converter/1 -> Divide1/1, MATLAB Function1/5(velo)
  i/1 -> MATLAB Function/4(i), MATLAB Function1/6(i)
  connections:
  cable connection dist&velo/RConn3 -- PS-Simulink Converter/LConn1
  cable connection dist&velo/RConn1 -- Internal Force/RConn1 -- F/RConn1
  cable connection dist&velo/RConn2 -- PS-Simulink Converter4/LConn1
  Simulink-PS Converter1/RConn1 -- Internal Force/LConn2
  cable connection dist&velo/LConn1 -- B/RConn1 -- Internal Force/LConn1

== system dvoupatrak_15lan/Tensegrity tower/Cables/i-th cable force7 ==
  i : Inport
  l0 : Inport  Port=2
  Constant : Constant  Value=kp
  Constant1 : Constant  Value=bs
  Constant2 : Constant  Value=0
  Constant3 : Constant  Value=ks
  Constant4 : Constant  Value=bp
  Constant5 : Constant  Value=l0_init
  Divide : Product  Inputs=*/*
  Divide1 : Product  Inputs=**/
  Gain : Gain  Gain=-1
  Internal Force : sm_lib/Forces and Torques/Internal Force
      settings: SourceProductBaseCode=MS
  MATLAB Function : MATLAB Function  TreatAsAtomicUnit=on
  MATLAB Function1 : MATLAB Function  TreatAsAtomicUnit=on
  PS-Simulink Converter : nesl_utility/PS-Simulink Converter  PhysicalDomain=network_engine_domain  SubClassName=ps_output  LeftPortType=input  RightPortType=output  PseudoPeriodic=off  Frequencies=[]  Unit=inherit  AffineConversion=off
  PS-Simulink Converter4 : nesl_utility/PS-Simulink Converter  PhysicalDomain=network_engine_domain  SubClassName=ps_output  LeftPortType=input  RightPortType=output  PseudoPeriodic=off  Frequencies=[]  Unit=inherit  AffineConversion=off
  Simulink-PS Converter1 : nesl_utility/Simulink-PS Converter  PhysicalDomain=network_engine_domain  SubClassName=ps_input  LeftPortType=input  RightPortType=output  PseudoPeriodic=off  Frequencies=[]  NoiseDistribution=none  NoiseParameters=[]  Unit=1  AffineConversion=off  FilteringAndDerivatives=provide  SimscapeFilterOrder=1  InputFilterTimeConstant=0.001  UdotUserProvided=0
  Sum : Sum  Inputs=+++
  Switch : Switch
  Switch1 : Switch
  cable connection dist&velo : sm_lib/Frames and Transforms/Transform Sensor  MeasurementFrame=World  SenseAngle=off  SenseAxis=off  SenseAngle1=off  SenseAngle2=off  SenseAngle3=off  SenseQ=off  SenseR=off  SenseOmegaX=off  SenseOmegaY=off  SenseOmegaZ=off  SenseOmega1=off  SenseOmega2=off  SenseOmega3=off  SenseQDot=off  SenseRDot=off  SenseAlphaX=off  SenseAlphaY=off  SenseAlphaZ=off  SenseAlpha1=off  SenseAlpha2=off  SenseAlpha3=off  SenseQDDot=off  SenseRDDot=off  SenseX=off  SenseY=off  SenseZ=off  SenseRad=off  SenseAzim=off  SenseDist=on  SenseInc=off  SenseXDot=off  SenseYDot=off  SenseZDot=off  SenseRadDot=off  SenseAzimDot=off  SenseDistDot=on  SenseIncDot=off  SenseXDDot=off  SenseYDDot=off  SenseZDDot=off  SenseRadDDot=off  SenseAzimDDot=off  SenseDistDDot=off  SenseIncDDot=off
  li-l0i : Sum  Inputs=+-
  F : PMIOPort  Side=Right
  B : PMIOPort  Port=2  Side=Left
  wires:
  Constant1/1 -> MATLAB Function/2(bs)
  Switch1/1 -> Sum/3  "cable_linear_kinetic_damping"
  Divide/1 -> Switch/1
  Switch/1 -> Sum/2  "cable_elastic_force"
  MATLAB Function/2(bsi) -> Divide1/2
  Constant3/1 -> MATLAB Function/1(ks)
  Divide1/1 -> Switch1/1
  MATLAB Function/1(ksi) -> Divide/1
  Constant/1 -> MATLAB Function1/1(kp)
  Constant4/1 -> MATLAB Function1/2(bp)
  Constant5/1 -> MATLAB Function1/3(l0_init)
  MATLAB Function1/1(Fp) -> Sum/1  "parallel_spring_force"
  Sum/1 -> Gain/1
  Gain/1 -> Simulink-PS Converter1/1
  li-l0i/1 -> Switch/2, Divide/3, Switch1/2
  l0/1 -> MATLAB Function/3(l0)
  Constant2/1 -> Switch1/3, Switch/3
  MATLAB Function/3(l0i) -> Divide1/3, Divide/2, li-l0i/2
  PS-Simulink Converter4/1 -> li-l0i/1, MATLAB Function1/4(dist)
  PS-Simulink Converter/1 -> Divide1/1, MATLAB Function1/5(velo)
  i/1 -> MATLAB Function/4(i), MATLAB Function1/6(i)
  connections:
  cable connection dist&velo/RConn3 -- PS-Simulink Converter/LConn1
  cable connection dist&velo/RConn1 -- Internal Force/RConn1 -- F/RConn1
  cable connection dist&velo/RConn2 -- PS-Simulink Converter4/LConn1
  Simulink-PS Converter1/RConn1 -- Internal Force/LConn2
  cable connection dist&velo/LConn1 -- B/RConn1 -- Internal Force/LConn1

== system dvoupatrak_15lan/Tensegrity tower/Cables/i-th cable force8 ==
  i : Inport
  l0 : Inport  Port=2
  Constant : Constant  Value=kp
  Constant1 : Constant  Value=bs
  Constant2 : Constant  Value=0
  Constant3 : Constant  Value=ks
  Constant4 : Constant  Value=bp
  Constant5 : Constant  Value=l0_init
  Divide : Product  Inputs=*/*
  Divide1 : Product  Inputs=**/
  Gain : Gain  Gain=-1
  Internal Force : sm_lib/Forces and Torques/Internal Force
      settings: SourceProductBaseCode=MS
  MATLAB Function : MATLAB Function  TreatAsAtomicUnit=on
  MATLAB Function1 : MATLAB Function  TreatAsAtomicUnit=on
  PS-Simulink Converter : nesl_utility/PS-Simulink Converter  PhysicalDomain=network_engine_domain  SubClassName=ps_output  LeftPortType=input  RightPortType=output  PseudoPeriodic=off  Frequencies=[]  Unit=inherit  AffineConversion=off
  PS-Simulink Converter4 : nesl_utility/PS-Simulink Converter  PhysicalDomain=network_engine_domain  SubClassName=ps_output  LeftPortType=input  RightPortType=output  PseudoPeriodic=off  Frequencies=[]  Unit=inherit  AffineConversion=off
  Simulink-PS Converter1 : nesl_utility/Simulink-PS Converter  PhysicalDomain=network_engine_domain  SubClassName=ps_input  LeftPortType=input  RightPortType=output  PseudoPeriodic=off  Frequencies=[]  NoiseDistribution=none  NoiseParameters=[]  Unit=1  AffineConversion=off  FilteringAndDerivatives=provide  SimscapeFilterOrder=1  InputFilterTimeConstant=0.001  UdotUserProvided=0
  Sum : Sum  Inputs=+++
  Switch : Switch
  Switch1 : Switch
  cable connection dist&velo : sm_lib/Frames and Transforms/Transform Sensor  MeasurementFrame=World  SenseAngle=off  SenseAxis=off  SenseAngle1=off  SenseAngle2=off  SenseAngle3=off  SenseQ=off  SenseR=off  SenseOmegaX=off  SenseOmegaY=off  SenseOmegaZ=off  SenseOmega1=off  SenseOmega2=off  SenseOmega3=off  SenseQDot=off  SenseRDot=off  SenseAlphaX=off  SenseAlphaY=off  SenseAlphaZ=off  SenseAlpha1=off  SenseAlpha2=off  SenseAlpha3=off  SenseQDDot=off  SenseRDDot=off  SenseX=off  SenseY=off  SenseZ=off  SenseRad=off  SenseAzim=off  SenseDist=on  SenseInc=off  SenseXDot=off  SenseYDot=off  SenseZDot=off  SenseRadDot=off  SenseAzimDot=off  SenseDistDot=on  SenseIncDot=off  SenseXDDot=off  SenseYDDot=off  SenseZDDot=off  SenseRadDDot=off  SenseAzimDDot=off  SenseDistDDot=off  SenseIncDDot=off
  li-l0i : Sum  Inputs=+-
  F : PMIOPort  Side=Right
  B : PMIOPort  Port=2  Side=Left
  wires:
  Constant1/1 -> MATLAB Function/2(bs)
  Switch1/1 -> Sum/3  "cable_linear_kinetic_damping"
  Divide/1 -> Switch/1
  Switch/1 -> Sum/2  "cable_elastic_force"
  MATLAB Function/2(bsi) -> Divide1/2
  Constant3/1 -> MATLAB Function/1(ks)
  Divide1/1 -> Switch1/1
  MATLAB Function/1(ksi) -> Divide/1
  Constant/1 -> MATLAB Function1/1(kp)
  Constant4/1 -> MATLAB Function1/2(bp)
  Constant5/1 -> MATLAB Function1/3(l0_init)
  MATLAB Function1/1(Fp) -> Sum/1  "parallel_spring_force"
  Sum/1 -> Gain/1
  Gain/1 -> Simulink-PS Converter1/1
  li-l0i/1 -> Switch/2, Divide/3, Switch1/2
  l0/1 -> MATLAB Function/3(l0)
  Constant2/1 -> Switch1/3, Switch/3
  MATLAB Function/3(l0i) -> Divide1/3, Divide/2, li-l0i/2
  PS-Simulink Converter4/1 -> li-l0i/1, MATLAB Function1/4(dist)
  PS-Simulink Converter/1 -> Divide1/1, MATLAB Function1/5(velo)
  i/1 -> MATLAB Function/4(i), MATLAB Function1/6(i)
  connections:
  cable connection dist&velo/RConn3 -- PS-Simulink Converter/LConn1
  cable connection dist&velo/RConn1 -- Internal Force/RConn1 -- F/RConn1
  cable connection dist&velo/RConn2 -- PS-Simulink Converter4/LConn1
  Simulink-PS Converter1/RConn1 -- Internal Force/LConn2
  cable connection dist&velo/LConn1 -- B/RConn1 -- Internal Force/LConn1

== system dvoupatrak_15lan/Tensegrity tower/Cables/i-th cable force9 ==
  i : Inport
  l0 : Inport  Port=2
  Constant : Constant  Value=kp
  Constant1 : Constant  Value=bs
  Constant2 : Constant  Value=0
  Constant3 : Constant  Value=ks
  Constant4 : Constant  Value=bp
  Constant5 : Constant  Value=l0_init
  Divide : Product  Inputs=*/*
  Divide1 : Product  Inputs=**/
  Gain : Gain  Gain=-1
  Internal Force : sm_lib/Forces and Torques/Internal Force
      settings: SourceProductBaseCode=MS
  MATLAB Function : MATLAB Function  TreatAsAtomicUnit=on
  MATLAB Function1 : MATLAB Function  TreatAsAtomicUnit=on
  PS-Simulink Converter : nesl_utility/PS-Simulink Converter  PhysicalDomain=network_engine_domain  SubClassName=ps_output  LeftPortType=input  RightPortType=output  PseudoPeriodic=off  Frequencies=[]  Unit=inherit  AffineConversion=off
  PS-Simulink Converter4 : nesl_utility/PS-Simulink Converter  PhysicalDomain=network_engine_domain  SubClassName=ps_output  LeftPortType=input  RightPortType=output  PseudoPeriodic=off  Frequencies=[]  Unit=inherit  AffineConversion=off
  Simulink-PS Converter1 : nesl_utility/Simulink-PS Converter  PhysicalDomain=network_engine_domain  SubClassName=ps_input  LeftPortType=input  RightPortType=output  PseudoPeriodic=off  Frequencies=[]  NoiseDistribution=none  NoiseParameters=[]  Unit=1  AffineConversion=off  FilteringAndDerivatives=provide  SimscapeFilterOrder=1  InputFilterTimeConstant=0.001  UdotUserProvided=0
  Sum : Sum  Inputs=+++
  Switch : Switch
  Switch1 : Switch
  cable connection dist&velo : sm_lib/Frames and Transforms/Transform Sensor  MeasurementFrame=World  SenseAngle=off  SenseAxis=off  SenseAngle1=off  SenseAngle2=off  SenseAngle3=off  SenseQ=off  SenseR=off  SenseOmegaX=off  SenseOmegaY=off  SenseOmegaZ=off  SenseOmega1=off  SenseOmega2=off  SenseOmega3=off  SenseQDot=off  SenseRDot=off  SenseAlphaX=off  SenseAlphaY=off  SenseAlphaZ=off  SenseAlpha1=off  SenseAlpha2=off  SenseAlpha3=off  SenseQDDot=off  SenseRDDot=off  SenseX=off  SenseY=off  SenseZ=off  SenseRad=off  SenseAzim=off  SenseDist=on  SenseInc=off  SenseXDot=off  SenseYDot=off  SenseZDot=off  SenseRadDot=off  SenseAzimDot=off  SenseDistDot=on  SenseIncDot=off  SenseXDDot=off  SenseYDDot=off  SenseZDDot=off  SenseRadDDot=off  SenseAzimDDot=off  SenseDistDDot=off  SenseIncDDot=off
  li-l0i : Sum  Inputs=+-
  F : PMIOPort  Side=Right
  B : PMIOPort  Port=2  Side=Left
  wires:
  Constant1/1 -> MATLAB Function/2(bs)
  Switch1/1 -> Sum/3  "cable_linear_kinetic_damping"
  Divide/1 -> Switch/1
  Switch/1 -> Sum/2  "cable_elastic_force"
  MATLAB Function/2(bsi) -> Divide1/2
  Constant3/1 -> MATLAB Function/1(ks)
  Divide1/1 -> Switch1/1
  MATLAB Function/1(ksi) -> Divide/1
  Constant/1 -> MATLAB Function1/1(kp)
  Constant4/1 -> MATLAB Function1/2(bp)
  Constant5/1 -> MATLAB Function1/3(l0_init)
  MATLAB Function1/1(Fp) -> Sum/1  "parallel_spring_force"
  Sum/1 -> Gain/1
  Gain/1 -> Simulink-PS Converter1/1
  li-l0i/1 -> Switch/2, Divide/3, Switch1/2
  l0/1 -> MATLAB Function/3(l0)
  Constant2/1 -> Switch1/3, Switch/3
  MATLAB Function/3(l0i) -> Divide1/3, Divide/2, li-l0i/2
  PS-Simulink Converter4/1 -> li-l0i/1, MATLAB Function1/4(dist)
  PS-Simulink Converter/1 -> Divide1/1, MATLAB Function1/5(velo)
  i/1 -> MATLAB Function/4(i), MATLAB Function1/6(i)
  connections:
  cable connection dist&velo/RConn3 -- PS-Simulink Converter/LConn1
  cable connection dist&velo/RConn1 -- Internal Force/RConn1 -- F/RConn1
  cable connection dist&velo/RConn2 -- PS-Simulink Converter4/LConn1
  Simulink-PS Converter1/RConn1 -- Internal Force/LConn2
  cable connection dist&velo/LConn1 -- B/RConn1 -- Internal Force/LConn1

== system dvoupatrak_15lan/Tensegrity tower/Excitation Subsystem/Cluster of Random Oscillators <0,1> ==
  freq : Inport
  Mux : Mux  Inputs=15
  Rand Oscillator 1 : Subsystem
  Rand Oscillator 10 : Subsystem
  Rand Oscillator 11 : Subsystem
  Rand Oscillator 12 : Subsystem
  Rand Oscillator 13 : Subsystem
  Rand Oscillator 14 : Subsystem
  Rand Oscillator 15 : Subsystem
  Rand Oscillator 2 : Subsystem
  Rand Oscillator 3 : Subsystem
  Rand Oscillator 4 : Subsystem
  Rand Oscillator 5 : Subsystem
  Rand Oscillator 6 : Subsystem
  Rand Oscillator 7 : Subsystem
  Rand Oscillator 8 : Subsystem
  Rand Oscillator 9 : Subsystem
  out : Outport
  wires:
  Rand Oscillator 2/1(Out1) -> Mux/2
  Rand Oscillator 5/1(Out1) -> Mux/5
  Rand Oscillator 3/1(Out1) -> Mux/3
  Rand Oscillator 6/1(Out1) -> Mux/6
  Rand Oscillator 7/1(Out1) -> Mux/7
  freq/1 -> Rand Oscillator 1/1(freq), Rand Oscillator 2/1(freq), Rand Oscillator 3/1(freq), Rand Oscillator 4/1(freq), Rand Oscillator 5/1(freq), Rand Oscillator 6/1(freq), Rand Oscillator 7/1(freq), Rand Oscillator 8/1(freq), Rand Oscillator 9/1(freq), Rand Oscillator 10/1(freq), Rand Oscillator 12/1(freq), Rand Oscillator 13/1(freq), Rand Oscillator 14/1(freq), Rand Oscillator 15/1(freq), Rand Oscillator 11/1(freq)
  Rand Oscillator 1/1(Out1) -> Mux/1
  Rand Oscillator 4/1(Out1) -> Mux/4
  Rand Oscillator 11/1(Out1) -> Mux/11
  Rand Oscillator 8/1(Out1) -> Mux/8
  Rand Oscillator 14/1(Out1) -> Mux/14
  Rand Oscillator 13/1(Out1) -> Mux/13
  Rand Oscillator 10/1(Out1) -> Mux/10
  Rand Oscillator 12/1(Out1) -> Mux/12
  Rand Oscillator 9/1(Out1) -> Mux/9
  Rand Oscillator 15/1(Out1) -> Mux/15
  Mux/1 -> out/1

== system dvoupatrak_15lan/Tensegrity tower/Excitation Subsystem/Cluster of Random Oscillators <0,1>/Rand Oscillator 1 ==
  freq : Inport
  Uniform Random Number : UniformRandomNumber  Minimum=0  SampleTime=0.1
  Varying Lowpass Filter : cstblocks/Linear Parameter Varying/Varying Lowpass Filter  N=2
      settings: SourceProductName=Control System Toolbox
  Out1 : Outport
  wires:
  Uniform Random Number/1 -> Varying Lowpass Filter/1
  freq/1 -> Varying Lowpass Filter/2
  Varying Lowpass Filter/1 -> Out1/1

== system dvoupatrak_15lan/Tensegrity tower/Excitation Subsystem/Cluster of Random Oscillators <0,1>/Rand Oscillator 10 ==
  freq : Inport
  Uniform Random Number : UniformRandomNumber  Minimum=0  Seed=10  SampleTime=0.1
  Varying Lowpass Filter : cstblocks/Linear Parameter Varying/Varying Lowpass Filter  N=2
      settings: SourceProductName=Control System Toolbox
  Out1 : Outport
  wires:
  Varying Lowpass Filter/1 -> Out1/1
  freq/1 -> Varying Lowpass Filter/2
  Uniform Random Number/1 -> Varying Lowpass Filter/1

== system dvoupatrak_15lan/Tensegrity tower/Excitation Subsystem/Cluster of Random Oscillators <0,1>/Rand Oscillator 11 ==
  freq : Inport
  Uniform Random Number : UniformRandomNumber  Minimum=0  Seed=11  SampleTime=0.1
  Varying Lowpass Filter : cstblocks/Linear Parameter Varying/Varying Lowpass Filter  N=2
      settings: SourceProductName=Control System Toolbox
  Out1 : Outport
  wires:
  Uniform Random Number/1 -> Varying Lowpass Filter/1
  freq/1 -> Varying Lowpass Filter/2
  Varying Lowpass Filter/1 -> Out1/1

== system dvoupatrak_15lan/Tensegrity tower/Excitation Subsystem/Cluster of Random Oscillators <0,1>/Rand Oscillator 12 ==
  freq : Inport
  Uniform Random Number : UniformRandomNumber  Minimum=0  Seed=12  SampleTime=0.1
  Varying Lowpass Filter : cstblocks/Linear Parameter Varying/Varying Lowpass Filter  N=2
      settings: SourceProductName=Control System Toolbox
  Out1 : Outport
  wires:
  Varying Lowpass Filter/1 -> Out1/1
  freq/1 -> Varying Lowpass Filter/2
  Uniform Random Number/1 -> Varying Lowpass Filter/1

== system dvoupatrak_15lan/Tensegrity tower/Excitation Subsystem/Cluster of Random Oscillators <0,1>/Rand Oscillator 13 ==
  freq : Inport
  Uniform Random Number : UniformRandomNumber  Minimum=0  Seed=13  SampleTime=0.1
  Varying Lowpass Filter : cstblocks/Linear Parameter Varying/Varying Lowpass Filter  N=2
      settings: SourceProductName=Control System Toolbox
  Out1 : Outport
  wires:
  Uniform Random Number/1 -> Varying Lowpass Filter/1
  freq/1 -> Varying Lowpass Filter/2
  Varying Lowpass Filter/1 -> Out1/1
